simulink model "automobilKocenjeBrzinaUdaljenostSimulink2012B"  (R2012b)
settings: Solver=ode45  SolverMode=SingleTasking  StartTime=0.0  StopTime=10.0  RelTol=1e-3
libraries: simulink x2, fuzblock x1
settings Model: CovMetricSettings=dwe  CovHtmlReporting=off  covSaveCumulativeToWorkspaceVar=off  CovSaveSingleToWorkspaceVar=off  CovExternalEMLEnable=on  Creator=Hp  LastModifiedBy=Aldin
settings DataIOCC: LimitDataPoints=off  SaveFormat=StructureWithTime  ReturnWorkspaceOutputs=on
settings OptimizationCC: ExpressionDepthLimit=128
settings DebuggingCC: UnderspecifiedInitializationDetection=Simplified  MergeDetectMultiDrivingBlocksExec=error  SolverPrmCheckMsg=none  FrameProcessingCompatibilityMsg=error  StateNameClashWarn=none  SFUnexpectedBacktrackingDiag=error  SFNoUnconditionalDefaultTransitionDiag=error
settings HardwareCC: ProdBitPerPointer=64  ProdLargestAtomicFloat=Float  ProdIntDivRoundTo=Zero  ProdEndianess=LittleEndian  ProdHWDeviceType=Specified
settings ModelReferenceCC: PropagateSignalLabelsOutOfModel=on
settings SFSimCC: SimUseLocalCustomCode=on
settings RTWCC: RTWUseLocalCustomCode=on
settings CodeAppCC: CustomSymbolStrType=$N$R$M_T
settings GRTTargetCC: CodeReplacementLibrary=C99 (ISO)

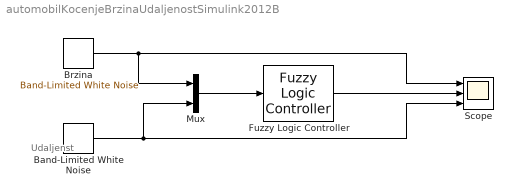
== system automobilKocenjeBrzinaUdaljenostSimulink2012B ==
  note: Udaljenst
  Band-Limited White Noise : simulink/Sources/Band-Limited White Noise  Cov=[150]  Ts=0.1  seed=[23341]
  Brzina : simulink/Sources/Band-Limited White Noise  Cov=[100]  Ts=0.1  seed=[23341]
  Fuzzy Logic Controller : fuzblock/Fuzzy Logic  Controller  FIS=automobilKocenjeBrzinaUdaljenost
  Mux : Mux  Inputs=2
  Scope : Scope  NumInputPorts=3
      settings: TimeRange=auto  MaxDataPoints=5000  SaveToWorkspace=off  SaveName=ScopeData  YMin=-113.9215~-5~-5  YMax=145.71139~5~5  SampleTime=-1
  wires:
  Mux/1 -> Fuzzy Logic Controller/1
  Brzina/1 -> Scope/1, Mux/1
  Band-Limited White Noise/1 -> Scope/3, Mux/2
  Fuzzy Logic Controller/1 -> Scope/2
